simulink model "red_beob1"  (Simulink 4.00)
settings: Solver=ode45  StartTime=0.0  StopTime=10  RelTol=1e-3
values from neighbouring files (symbols this model uses):
  A21 = A(n1+1:n, 1:n1)    [red_beob_1.m]
  A22 = A(n1+1:n, n1+1:n)    [red_beob_1.m]
  ausgang = [zeros(mo, n1), eye(mo,mo)]    [red_beob_1.m]
  B2 = B(n1+1:n,1:mi)    [red_beob_1.m]
  C = [Cp, zeros(1,ns)]    [akalm1.m]    (also in kalm1.m = my_sys1.c; kalm2.m = my_sys1.c; kalm3.m = my_sys1.c; kalm4.m = [eye(3,3), zeros(3,3)])
  D = [0]    [akalm1.m]    (also in kalm1.m = my_sys1.d; kalm2.m = my_sys1.d; kalm3.m = my_sys1.d; kalm4.m = zeros(3,3))
  Ke = K'    [abeob1.m]    (also in estimate_1.m = place(a', c', p).'; estimate_2.m = place(a', c', p).'; estimate_3.m = place(a', c', p).'; estimate_31.m = place(a', c', p).')
  mess_zust = [eye(n1,n1), zeros(n1, mo)]    [red_beob_1.m]
  mi = 3    [red_beob_1.m]
  n = length(t)    [plot_mt.m]    (also in red_beob_1.m = 6)
libraries: simulink3 x1, cstblocks x1
settings Model: LastModifiedBy=Administrator  BlockReductionOpt=off

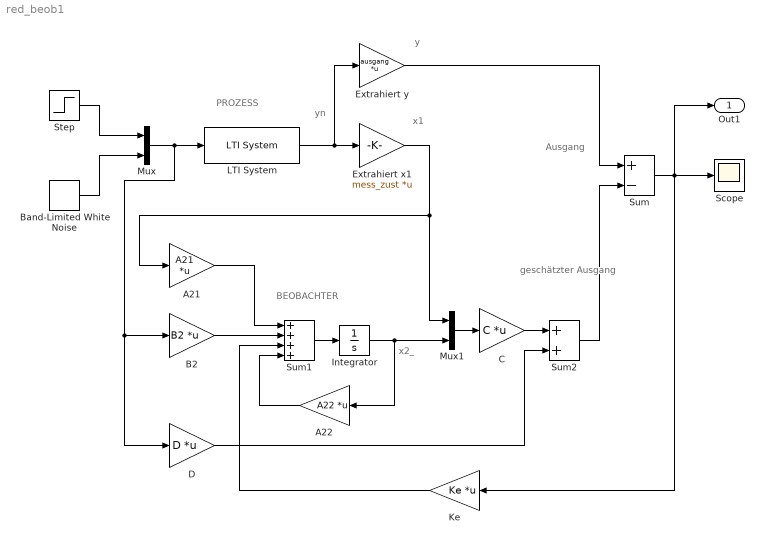
== system red_beob1 ==
  note: yn
  note: x1
  note: y
  note: x2_
  note: BEOBACHTER
  note: PROZESS
  note: geschätzter
      | Ausgang
  note: Ausgang
  A21 : Gain  Gain=A21  Multiplication=Matrix(K*u)  SaturateOnIntegerOverflow=on
  A22 : Gain  Orientation=left  Gain=A22  Multiplication=Matrix(K*u)  SaturateOnIntegerOverflow=on
  B2 : Gain  Gain=B2  Multiplication=Matrix(K*u)  SaturateOnIntegerOverflow=on
  Band-Limited White Noise : simulink3/Sources/Band-Limited White Noise  Cov=[0.01]  Ts=0.01  seed=[23341]
  C : Gain  Gain=C  Multiplication=Matrix(K*u)  SaturateOnIntegerOverflow=on
  D : Gain  Gain=D  Multiplication=Matrix(K*u)  SaturateOnIntegerOverflow=on
  Extrahiert x1 : Gain  Gain=mess_zust  Multiplication=Matrix(K*u)  SaturateOnIntegerOverflow=on
  Extrahiert y : Gain  Gain=ausgang  Multiplication=Matrix(K*u)  SaturateOnIntegerOverflow=on
  Integrator : Integrator  ExternalReset=none  InitialConditionSource=internal  InitialCondition=0  LimitOutput=off  UpperSaturationLimit=inf  LowerSaturationLimit=-inf  ShowSaturationPort=off  ShowStatePort=off  AbsoluteTolerance=auto
  Ke : Gain  Orientation=left  Gain=Ke  Multiplication=Matrix(K*u)  SaturateOnIntegerOverflow=on
  LTI System : cstblocks/LTI System  sys=my_sys_n  IC=randn(1,n)
  Mux : Mux  Inputs=2
  Mux1 : Mux  Inputs=2
  Scope : Scope
      settings: TimeRange=auto  YMin=-5  YMax=5  SaveToWorkspace=off  SaveName=ScopeData  LimitDataPoints=on  MaxDataPoints=5000
  Step : Step  Time=0  Before=0  After=ones(1, mi-1)  SampleTime=0
  Sum : Sum  Inputs=+-  SaturateOnIntegerOverflow=on
  Sum1 : Sum  Inputs=++++  SaturateOnIntegerOverflow=on
  Sum2 : Sum  Inputs=++  SaturateOnIntegerOverflow=on
  Out1 : Outport  Port=1
  wires:
  LTI System/1 -> Extrahiert x1/1, Extrahiert y/1
  Mux/1 -> LTI System/1, B2/1, D/1
  Step/1 -> Mux/1
  Band-Limited White Noise/1 -> Mux/2
  Extrahiert x1/1 -> Mux1/1, A21/1
  Integrator/1 -> Mux1/2, A22/1
  Mux1/1 -> C/1
  Extrahiert y/1 -> Sum/1
  Sum/1 -> Scope/1, Ke/1, Out1/1
  Sum1/1 -> Integrator/1
  A21/1 -> Sum1/1
  B2/1 -> Sum1/2
  Ke/1 -> Sum1/3
  A22/1 -> Sum1/4
  C/1 -> Sum2/1
  Sum2/1 -> Sum/2
  D/1 -> Sum2/2
